simulink library "PositionSmoothener"  (R2016b)
settings: Solver=VariableStepAuto  StartTime=0.0  StopTime=10.0  RelTol=1e-3
undefined symbols (not defined in the file or in its folder): maxHomeAcceleration, maxHomeVelocity
libraries: PositionSmoothener x11, VariousLibrary x6, GaitHandler x2
settings Model: Creator=snyke7  LastModifiedBy=snyke7

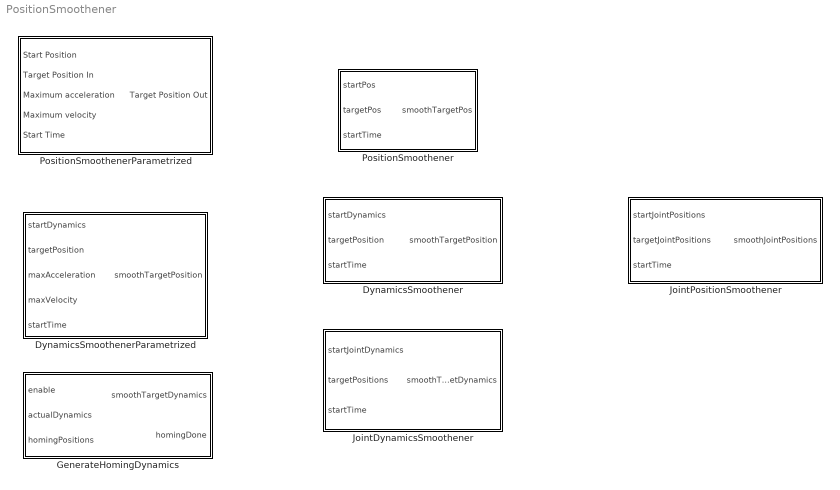
== system PositionSmoothener ==
  DynamicsSmoothener : Subsystem
  DynamicsSmoothenerParametrized : Subsystem
  GenerateHomingDynamics : Subsystem
  JointDynamicsSmoothener : Subsystem
  JointPositionSmoothener : Subsystem
  PositionSmoothener : Subsystem
  PositionSmoothenerParametrized : Subsystem

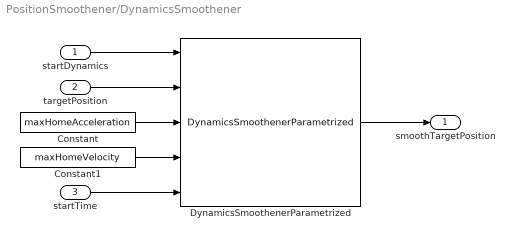
== system PositionSmoothener/DynamicsSmoothener ==
  startDynamics : Inport
  targetPosition : Inport  Port=2
  startTime : Inport  Port=3
  Constant : Constant  Value=maxHomeAcceleration
  Constant1 : Constant  Value=maxHomeVelocity
  DynamicsSmoothenerParametrized : PositionSmoothener/DynamicsSmoothenerParametrized
  smoothTargetPosition : Outport
  wires:
  targetPosition/1 -> DynamicsSmoothenerParametrized/2
  startDynamics/1 -> DynamicsSmoothenerParametrized/1
  startTime/1 -> DynamicsSmoothenerParametrized/5
  Constant1/1 -> DynamicsSmoothenerParametrized/4
  Constant/1 -> DynamicsSmoothenerParametrized/3
  DynamicsSmoothenerParametrized/1 -> smoothTargetPosition/1

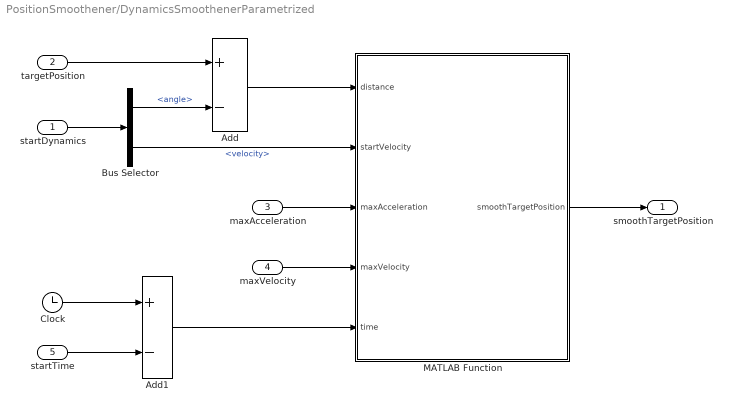
== system PositionSmoothener/DynamicsSmoothenerParametrized ==
  startDynamics : Inport
  targetPosition : Inport  Port=2
  maxAcceleration : Inport  Port=3
  maxVelocity : Inport  Port=4
  startTime : Inport  Port=5
  Add : Sum  Inputs=+-
  Add1 : Sum  Inputs=+-
  Bus Selector : BusSelector  OutputSignals=angle,velocity
  Clock : Clock
  MATLAB Function : MATLAB Function  TreatAsAtomicUnit=on
  smoothTargetPosition : Outport
  wires:
  MATLAB Function/1(smoothTargetPosition) -> smoothTargetPosition/1
  Add1/1 -> MATLAB Function/5(time)
  maxVelocity/1 -> MATLAB Function/4(maxVelocity)
  maxAcceleration/1 -> MATLAB Function/3(maxAcceleration)
  Bus Selector/2 -> MATLAB Function/2(startVelocity)  "<velocity>"
  Add/1 -> MATLAB Function/1(distance)
  startTime/1 -> Add1/2
  Clock/1 -> Add1/1
  Bus Selector/1 -> Add/2  "<angle>"
  targetPosition/1 -> Add/1
  startDynamics/1 -> Bus Selector/1

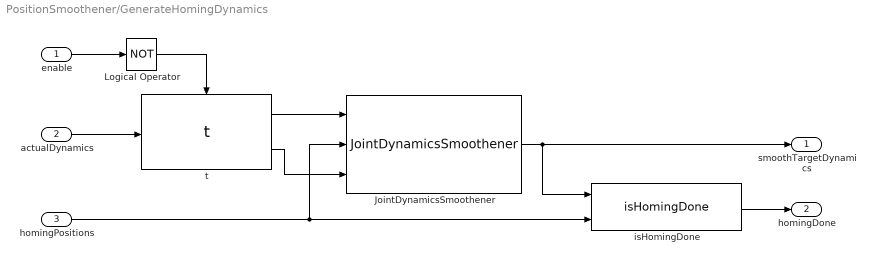
== system PositionSmoothener/GenerateHomingDynamics ==
  enable : Inport
  actualDynamics : Inport  Port=2
  homingPositions : Inport  Port=3
  JointDynamicsSmoothener : PositionSmoothener/JointDynamicsSmoothener
  Logical Operator : Logic  Operator=NOT  AllPortsSameDT=off  OutDataTypeStr=boolean
  isHomingDone : GaitHandler/GaitHandler/HomingGaitGenerator/Subsystem1/isHomingDone
  t : GaitHandler/GaitHandler/HomingGaitGenerator/Subsystem1/t
  smoothTargetDynamics : Outport
  homingDone : Outport  Port=2
  wires:
  Logical Operator/1 -> t/Enable
  enable/1 -> Logical Operator/1
  homingPositions/1 -> JointDynamicsSmoothener/2, isHomingDone/2
  actualDynamics/1 -> t/1
  isHomingDone/1 -> homingDone/1
  t/1 -> JointDynamicsSmoothener/1
  t/2 -> JointDynamicsSmoothener/3
  JointDynamicsSmoothener/1 -> smoothTargetDynamics/1, isHomingDone/1

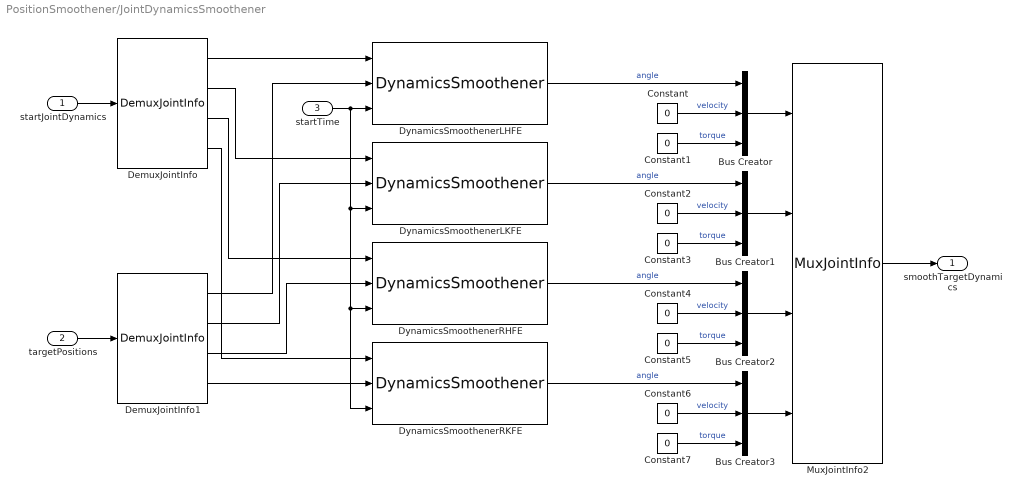
== system PositionSmoothener/JointDynamicsSmoothener ==
  startJointDynamics : Inport
  targetPositions : Inport  Port=2
  startTime : Inport  Port=3
  Bus Creator{,1..3} (4 alike) : BusCreator  Inputs=3  OutDataTypeStr=Bus: JointDynamics  NonVirtualBus=on
  Constant{,1..7} (8 alike) : Constant  Value=0
  DemuxJointInfo : VariousLibrary/DemuxJointInfo
  DemuxJointInfo1 : VariousLibrary/DemuxJointInfo
  DynamicsSmoothenerLHFE : PositionSmoothener/DynamicsSmoothener
  DynamicsSmoothenerLKFE : PositionSmoothener/DynamicsSmoothener
  DynamicsSmoothenerRHFE : PositionSmoothener/DynamicsSmoothener
  DynamicsSmoothenerRKFE : PositionSmoothener/DynamicsSmoothener
  MuxJointInfo2 : VariousLibrary/MuxJointInfo
  smoothTargetDynamics : Outport
  wires:
  startJointDynamics/1 -> DemuxJointInfo/1
  targetPositions/1 -> DemuxJointInfo1/1
  startTime/1 -> DynamicsSmoothenerRKFE/3, DynamicsSmoothenerRHFE/3, DynamicsSmoothenerLKFE/3, DynamicsSmoothenerLHFE/3
  DemuxJointInfo/1 -> DynamicsSmoothenerLHFE/1
  DemuxJointInfo/2 -> DynamicsSmoothenerLKFE/1
  DemuxJointInfo/3 -> DynamicsSmoothenerRHFE/1
  DemuxJointInfo/4 -> DynamicsSmoothenerRKFE/1
  DemuxJointInfo1/1 -> DynamicsSmoothenerLHFE/2
  DemuxJointInfo1/2 -> DynamicsSmoothenerLKFE/2
  DemuxJointInfo1/3 -> DynamicsSmoothenerRHFE/2
  DemuxJointInfo1/4 -> DynamicsSmoothenerRKFE/2
  Constant/1 -> Bus Creator/2  "velocity"
  Constant1/1 -> Bus Creator/3  "torque"
  Bus Creator/1 -> MuxJointInfo2/1
  Constant2/1 -> Bus Creator1/2  "velocity"
  Constant3/1 -> Bus Creator1/3  "torque"
  Bus Creator1/1 -> MuxJointInfo2/2
  Constant4/1 -> Bus Creator2/2  "velocity"
  Constant5/1 -> Bus Creator2/3  "torque"
  Bus Creator2/1 -> MuxJointInfo2/3
  Constant6/1 -> Bus Creator3/2  "velocity"
  Constant7/1 -> Bus Creator3/3  "torque"
  Bus Creator3/1 -> MuxJointInfo2/4
  DynamicsSmoothenerLHFE/1 -> Bus Creator/1  "angle"
  DynamicsSmoothenerLKFE/1 -> Bus Creator1/1  "angle"
  DynamicsSmoothenerRHFE/1 -> Bus Creator2/1  "angle"
  DynamicsSmoothenerRKFE/1 -> Bus Creator3/1  "angle"
  MuxJointInfo2/1 -> smoothTargetDynamics/1

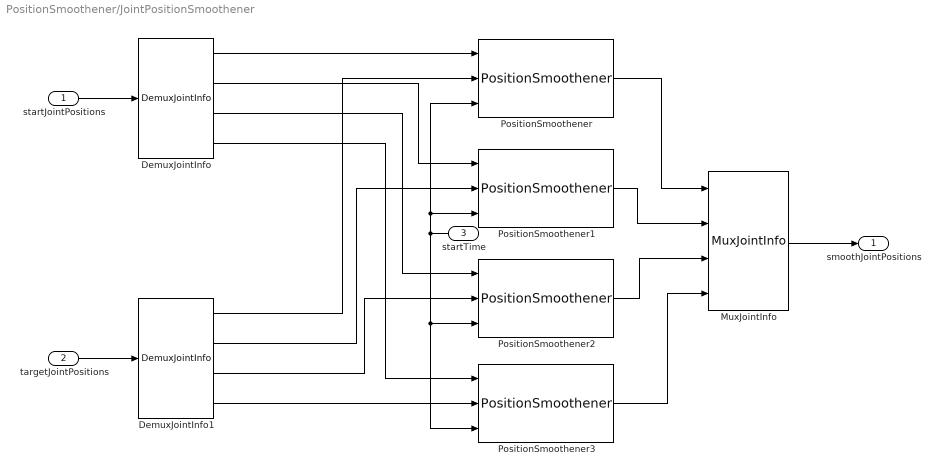
== system PositionSmoothener/JointPositionSmoothener ==
  startJointPositions : Inport
  targetJointPositions : Inport  Port=2
  startTime : Inport  Port=3
  DemuxJointInfo : VariousLibrary/DemuxJointInfo
  DemuxJointInfo1 : VariousLibrary/DemuxJointInfo
  MuxJointInfo : VariousLibrary/MuxJointInfo
  PositionSmoothener{,1..3} (4 alike) : PositionSmoothener/PositionSmoothener
  smoothJointPositions : Outport
  wires:
  startTime/1 -> PositionSmoothener2/3, PositionSmoothener3/3, PositionSmoothener/3, PositionSmoothener1/3
  startJointPositions/1 -> DemuxJointInfo/1
  targetJointPositions/1 -> DemuxJointInfo1/1
  DemuxJointInfo/1 -> PositionSmoothener/1
  DemuxJointInfo/2 -> PositionSmoothener1/1
  DemuxJointInfo/3 -> PositionSmoothener2/1
  DemuxJointInfo/4 -> PositionSmoothener3/1
  DemuxJointInfo1/4 -> PositionSmoothener3/2
  DemuxJointInfo1/3 -> PositionSmoothener2/2
  DemuxJointInfo1/2 -> PositionSmoothener1/2
  DemuxJointInfo1/1 -> PositionSmoothener/2
  PositionSmoothener/1 -> MuxJointInfo/1
  PositionSmoothener1/1 -> MuxJointInfo/2
  PositionSmoothener2/1 -> MuxJointInfo/3
  PositionSmoothener3/1 -> MuxJointInfo/4
  MuxJointInfo/1 -> smoothJointPositions/1

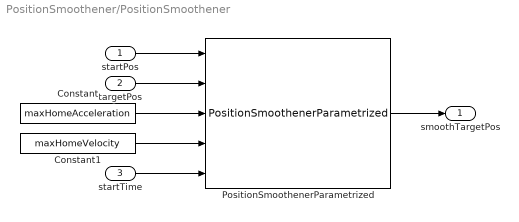
== system PositionSmoothener/PositionSmoothener ==
  startPos : Inport
  targetPos : Inport  Port=2
  startTime : Inport  Port=3
  Constant : Constant  Value=maxHomeAcceleration
  Constant1 : Constant  Value=maxHomeVelocity
  PositionSmoothenerParametrized : PositionSmoothener/PositionSmoothenerParametrized
  smoothTargetPos : Outport
  wires:
  startTime/1 -> PositionSmoothenerParametrized/5
  startPos/1 -> PositionSmoothenerParametrized/1
  targetPos/1 -> PositionSmoothenerParametrized/2
  Constant/1 -> PositionSmoothenerParametrized/3
  Constant1/1 -> PositionSmoothenerParametrized/4
  PositionSmoothenerParametrized/1 -> smoothTargetPos/1

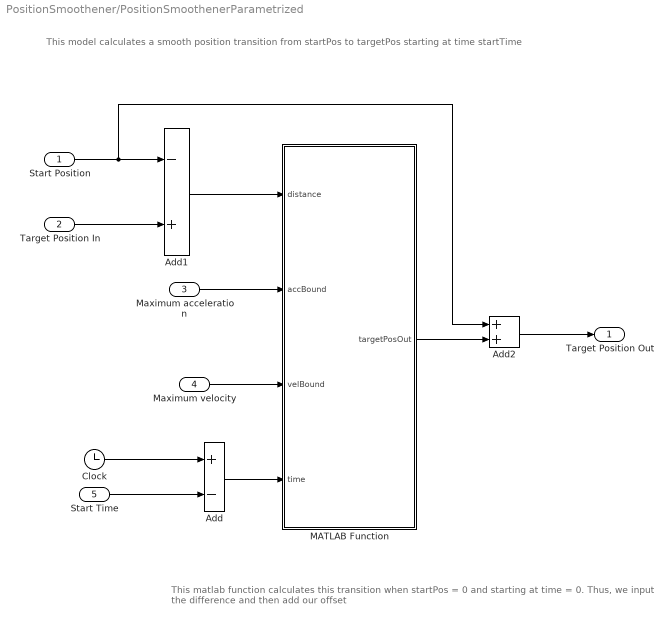
== system PositionSmoothener/PositionSmoothenerParametrized ==
  note: This matlab function calculates this transition when startPos = 0 and starting at time = 0. Thus, we input the difference and then add our offset
  note: This model calculates a smooth position transition from startPos to targetPos starting at time startTime
  Start Position : Inport
  Target Position In : Inport  Port=2
  Maximum acceleration : Inport  Port=3
  Maximum velocity : Inport  Port=4
  Start Time : Inport  Port=5
  Add : Sum  Inputs=+-
  Add1 : Sum  Inputs=-+
  Add2 : Sum
  Clock : Clock
  MATLAB Function : MATLAB Function  TreatAsAtomicUnit=on
  Target Position Out : Outport
  wires:
  Clock/1 -> Add/1
  Start Time/1 -> Add/2
  Target Position In/1 -> Add1/2
  Start Position/1 -> Add2/1, Add1/1
  Add1/1 -> MATLAB Function/1(distance)
  Maximum acceleration/1 -> MATLAB Function/2(accBound)
  Maximum velocity/1 -> MATLAB Function/3(velBound)
  Add/1 -> MATLAB Function/4(time)
  MATLAB Function/1(targetPosOut) -> Add2/2
  Add2/1 -> Target Position Out/1

== matlab function PositionSmoothener/PositionSmoothenerParametrized/MATLAB Function ==
  data: distance input; targetPosOut output; accBound input; velBound input; time input
function targetPosOut = getTargetPosOut(distance, accBound, velBound, time)
%% Calculates the value of a smooth transition from zero to distance at time
% Calculates the position value at time time of a smooth transition with
% maximum acceleration accBound and maximum velocity velBound
% A smooth transition is defined as arrival at the destination point with
% first derivative zero

% First, we see how long it would take to reach distance if we first
% accelerate as fast as possible and then decelerate as fast as possible
% This corresponds to p(t) = 0.5*a*t^2 untill we're halfway. Symmetry now
% takes care of reaching the destination with the desired properties. So we
% solve: 0.5*distance = 0.5*a*t^2
%       distance = a*t^2
%       t = sqrt(distance/a).
% This is the time to reach halfway so the total time needed is twice this.
% We also take the absolute value of the distance, as for negative distance
% we will use negative acceleration
timeNeeded = 2*sqrt(abs(distance)/accBound);

% To see if we can use the approach above, we check if the maximum velocity
% in this approach is higher than the velocity bound. We have
% v(t) = a*t for t <= timeNeeded/2 so the maximum velocity reached is:
maxVel = accBound*timeNeeded/2;

% note that we will correct for the sign of distance at the end of the
% function
if maxVel >= velBound 
    % In this case we have to speed up to the maximum allowed velocity,
    % then continue at a constant velocity untill we reach the point where
    % speeding down at the maximum deceleration stops us exactly at the
    % desired destination
    
    % We first calculate how long we can accelerate until we reach maximum
    % velocity. Since v(t) = at:
    timeToStopAcc = velBound/accBound;
    % The distance travelled in this time is equal to p(t) = 0.5*a*t^2
    distanceAcc = 0.5*accBound*timeToStopAcc^2;
    % Due to symmetry:
    distanceDec = distanceAcc;
    % Remaining distance to be travelled at constant velocity:
    distanceRem = abs(distance) - distanceAcc - distanceDec;
    % We now calculate the time we are at constant velocity with p(t) = vt
    timeConstantVel = distanceRem/velBound;
    % After acceleration and time at constantVel, we start decelerating:
    timeToStartDec = timeToStopAcc + timeConstantVel;
    % Finally, due to symmetry since deceleration takes the same amount of
    % time as acceleration:
    timeNeeded = timeToStartDec + timeToStopAcc;
    
    % Now we use the current time to calculate the targetPosOut.
    if time < timeToStopAcc
        % Now p(t) = 0.5 * a * t^2
        targetPosOut = 0.5 * accBound * time^2;
    elseif time < timeToStartDec
        % Then we have travelled distanceAcc, and the distance travelled at
        % constant velocity is given by p(t) = v(time - timeToStopAcc)
        travelledPos = distanceAcc;
        targetPosOut = travelledPos + velBound * (time - timeToStopAcc);
    else
        % Now we start decelerating. The travelled distance is given by
        % distanceAcc + distanceRem
        travelledPos = distanceAcc + distanceRem;
        % The velocity at a given time is equal to the maxvelocity minus
        % the acceleration times the time passed since timeToStartDec. The
        % position travelled since timeToStartDec is the integral from
        % timeToStartDec to time over this velocity. As we know the total
        % area is timeToStartAcc, we can calculate the desired area by
        % substracting the other part. That part is easy to calculate,
        % since it is the same distance as travelled when speeding up from
        % 0 to timeNeeded - time. So:
        targetPosOut = travelledPos + distanceDec - 0.5*accBound*(timeNeeded - time)^2;
    end
else
    % This means we can keep accelerating until halfway, then decelerate
    midTime = timeNeeded/2;
    if time < midTime
        % in the acceleration phase: p(t) = 0.5*a*t^2
        targetPosOut = 0.5 * accBound * time^2;
    else
        % Due to how we chose timeNeeded, we have travelled exactly half of
        % the distance
        travelledPos = abs(distance)/2;
        % Same reasoning as for the deceleration phase of the three-phase
        % way, but now distanceDec = abs(distance)/2 so that we have:
        targetPosOut = travelledPos + abs(distance)/2 - 0.5 * accBound*(timeNeeded - time)^2;
    end
end
if sign(distance) == -1
    % then negate the targetPosition, as all calculations have been done
    % with abs(distance)
    targetPosOut = -targetPosOut;
end

% finally, if time > timeNeeded (which has now correctly been set), then we
% have reached the target position
if time > timeNeeded
    targetPosOut = distance;
end
end

== matlab function PositionSmoothener/DynamicsSmoothenerParametrized/MATLAB Function ==
  data: distance input; smoothTargetPosition output; startVelocity input; maxAcceleration input; maxVelocity input; time input
function smoothTargetPosition = getSmoothTransitionTo(distance, startVelocity, maxAcceleration, maxVelocity, time)
% wrapper for getSmoothTransitionTo
smoothTargetPosition = getSmoothTransitionTo(distance, startVelocity, maxAcceleration, maxVelocity, time);
end
